simulink model "a4"  (Simulink 8.7)
settings: Solver=VariableStepAuto  StartTime=0.0  StopTime=10  RelTol=1e-3
settings Model: Creator=Birger  LastModifiedBy=Birger
settings DataIOCC: LimitDataPoints=off  SaveFormat=Dataset
settings DebuggingCC: UnderspecifiedInitializationDetection=Simplified  MergeDetectMultiDrivingBlocksExec=error
settings HardwareCC: ProdBitPerPointer=64  ProdLargestAtomicFloat=Float  ProdIntDivRoundTo=Zero  ProdEndianess=LittleEndian  ProdWordSize=64  ProdHWDeviceType=Intel->x86-64 (Windows64)
settings ModelReferenceCC: PropagateSignalLabelsOutOfModel=on
settings ConfigComp: CovModelRefEnable=off

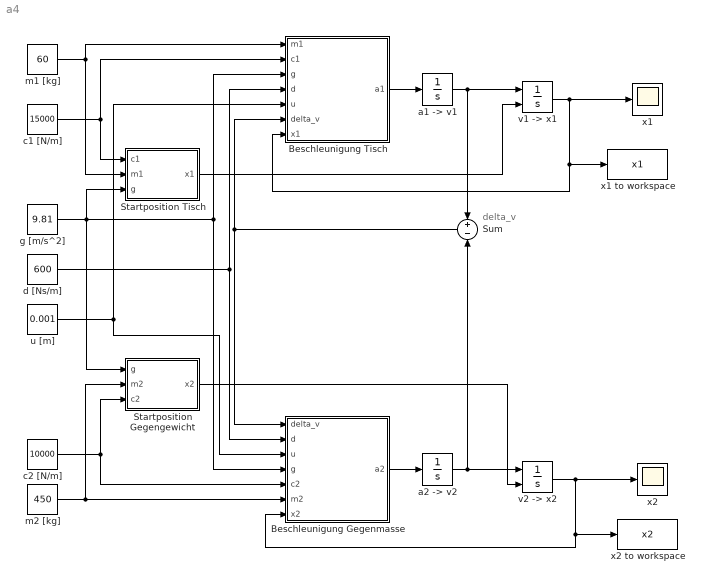
== system a4 ==
  note: delta_v
  Beschleunigung Gegenmasse : MATLAB Function  TreatAsAtomicUnit=on
  Beschleunigung Tisch : MATLAB Function  TreatAsAtomicUnit=on
  Startposition Gegengewicht : MATLAB Function  TreatAsAtomicUnit=on
  Startposition Tisch : MATLAB Function  TreatAsAtomicUnit=on
  Sum : Sum  Inputs=+-
  "a1 -> v1" : Integrator
  "a2 -> v2" : Integrator
  c1 [N/m] : Constant  Value=15000
  c2 [N/m] : Constant  Value=10000
  d [Ns/m] : Constant  Value=600
  g [m/s^2] : Constant  Value=9.81
  m1 [kg] : Constant  Value=60
  m2 [kg] : Constant  Value=450
  u [m] : Constant  Value=0.001
  "v1 -> x1" : Integrator  InitialConditionSource=external
  "v2 -> x2" : Integrator  InitialConditionSource=external
  x1 : Scope
  x1 to workspace : ToWorkspace  VariableName=x1  SaveFormat=Timeseries  SampleTime=-1
  x2 : Scope
  x2 to workspace : ToWorkspace  VariableName=x2  SaveFormat=Timeseries  SampleTime=-1
  wires:
  g [m/s^2]/1 -> Beschleunigung Gegenmasse/4(g), Beschleunigung Tisch/3(g), Startposition Gegengewicht/1(g), Startposition Tisch/3(g)
  m1 [kg]/1 -> Beschleunigung Tisch/1(m1), Startposition Tisch/2(m1)
  c1 [N/m]/1 -> Startposition Tisch/1(c1), Beschleunigung Tisch/2(c1)
  m2 [kg]/1 -> Beschleunigung Gegenmasse/6(m2), Startposition Gegengewicht/2(m2)
  c2 [N/m]/1 -> Startposition Gegengewicht/3(c2), Beschleunigung Gegenmasse/5(c2)
  d [Ns/m]/1 -> Beschleunigung Gegenmasse/2(d), Beschleunigung Tisch/4(d)
  u [m]/1 -> Beschleunigung Gegenmasse/3(u), Beschleunigung Tisch/5(u)
  Beschleunigung Tisch/1(a1) -> "a1 -> v1"/1
  "a1 -> v1"/1 -> "v1 -> x1"/1, Sum/1
  Startposition Tisch/1(x1) -> "v1 -> x1"/2
  "v1 -> x1"/1 -> x1/1, x1 to workspace/1, Beschleunigung Tisch/7(x1)
  Sum/1 -> Beschleunigung Gegenmasse/1(delta_v), Beschleunigung Tisch/6(delta_v)
  Beschleunigung Gegenmasse/1(a2) -> "a2 -> v2"/1
  "a2 -> v2"/1 -> "v2 -> x2"/1, Sum/2
  Startposition Gegengewicht/1(x2) -> "v2 -> x2"/2
  "v2 -> x2"/1 -> x2/1, Beschleunigung Gegenmasse/7(x2), x2 to workspace/1

== matlab function Startposition Gegengewicht ==
  data: g input double; x2 output double; m2 input double; c2 input double
function x2 = fcn(g,m2,c2)
%#codegen

x2 = -(m2*g) / (2*c2);

== matlab function Startposition Tisch ==
  data: c1 input double; m1 input double; g input double; x1 output double
function x1 = fcn(c1,m1,g)
%#codegen

x1 = -(m1*g) / (2*c1);

== matlab function Beschleunigung Tisch ==
  data: m1 input double; c1 input double; g input double; d input double; u input double; delta_v input double; a1 output double; x1 input double
function a1 = fcn(m1,c1,g,d,u,delta_v,x1)
%#codegen

delta_x1 = x1 - u;

Fg1 = m1 * g;
Fd = 2 * delta_v * d;
Fc1 = 2 * delta_x1 * c1;

a1 = (-Fg1 - Fd - Fc1)/m1;

== matlab function Beschleunigung Gegenmasse ==
  data: delta_v input double; d input double; u input double; g input double; c2 input double; m2 input double; a2 output double; x2 input double
function a2 = fcn(delta_v,d,u,g,c2,m2,x2)
%#codegen

delta_x2 = x2 - u;

Fg2 = m2 * g;
Fd = 2 * delta_v * d;
Fc2 = 2 * delta_x2 * c2;

a2 = (-Fg2 + Fd - Fc2)/m2;
